simulink model "test_motor_with_encoder"  (R2023b)
settings: Solver=ode4  StartTime=0.0  StopTime=10.0  FixedStep=ts  RelTol=1e-3  EnableMultiTasking=on
libraries: arduinolib x2, arduinosensorlib x1
settings Model: ExtModeTrigDuration=2  Creator=MunoLike  LastModifiedBy=MunoLike
settings OptimizationCC: EnhancedBackFolding=on  PassReuseOutputArgsAs=Individual arguments  ZeroExternalMemoryAtStartup=off  ZeroInternalMemoryAtStartup=off  MaxStackSize=64  OptimizeBlockOrder=speed  DifferentSizesBufferReuse=on  OptimizationCustomize=off  EfficientTunableParamExpr=on
settings DebuggingCC: ParameterTunabilityLossMsg=error
settings HardwareCC: ProdBitPerInt=16  ProdBitPerPointer=16  ProdBitPerSizeT=16  ProdBitPerPtrDiffT=16  ProdLargestAtomicFloat=None  ProdWordSize=8  ProdHWDeviceType=Atmel->AVR  UseEmbeddedCoderFeatures=off  UseSimulinkCoderFeatures=off
settings SFSimCC: MATLABDynamicMemAlloc=off
settings RTWCC: Description=Embedded Coder  SystemTargetFile=ert.tlc  HardwareBoard=Arduino Uno  TemplateMakefile=ert_default_tmf  Toolchain=Arduino AVR  BuildConfiguration=Faster Runs
settings CodeAppCC: ForceParamTrailComments=on  IgnoreCustomStorageClasses=off  OperatorAnnotations=on  SimulinkDataObjDesc=on  SFDataObjDesc=on  InsertBlockDesc=on
settings ERTTargetCC: SupportContinuousTime=on  SupportNonInlinedSFcns=on  SupportVariableSizeSignals=on  ExtModeTransport=3  ExtModeStaticAlloc=on  ExtModeAutomaticAllocSize=off  ExtModeStaticAllocSize=250  ExtModeMexFile=ext_xcp  ExtModeIntrfLevel=Level2 - Open

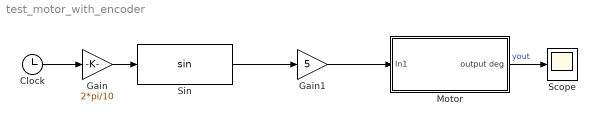
== system test_motor_with_encoder ==
  Clock : Clock
  Gain : Gain  Gain=2*pi/10
  Gain1 : Gain  Gain=5
  Motor : Subsystem
  Scope : Scope
  Sin : Trigonometry
  wires:
  Clock/1 -> Gain/1
  Motor/1(output deg) -> Scope/1  "yout"
  Gain/1 -> Sin/1
  Sin/1 -> Gain1/1
  Gain1/1 -> Motor/1(In1)

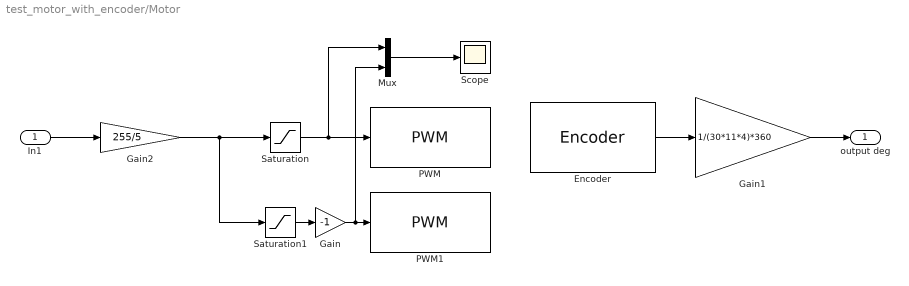
== system test_motor_with_encoder/Motor ==
  In1 : Inport  OutDataTypeStr=double
  Encoder : arduinosensorlib/Encoder  InputA=2  InputB=3  Mode=No reset  SampleTime=-1
  Gain : Gain  Gain=-1
  Gain1 : Gain  Gain=1/(30*11*4)*360  OutDataTypeStr=double
  Gain2 : Gain  Gain=255/5  ParamDataTypeStr=double  OutDataTypeStr=double
  Mux : Mux  Inputs=2
  PWM : arduinolib/PWM  pinNumber=5  frequencyType=Default  desiredFrequency=490.2  achievableFrequency=490.2
  PWM1 : arduinolib/PWM  pinNumber=6  frequencyType=Default  desiredFrequency=490.2  achievableFrequency=490.2
  Saturation : Saturate  UpperLimit=255  LowerLimit=0
  Saturation1 : Saturate  UpperLimit=0  LowerLimit=-255
  Scope : Scope
  output deg : Outport  OutDataTypeStr=double
  wires:
  In1/1 -> Gain2/1
  Saturation/1 -> Mux/1, PWM/1
  Saturation1/1 -> Gain/1
  Gain2/1 -> Saturation1/1, Saturation/1
  Gain1/1 -> output deg/1
  Encoder/1 -> Gain1/1
  Mux/1 -> Scope/1
  Gain/1 -> Mux/2, PWM1/1
